simulink model "lab3"  (R2019b)
settings: Solver=FixedStepAuto  StartTime=0.0  StopTime=100.0  RelTol=1e-3
settings Model: Creator=Michał  LastModifiedBy=Michał

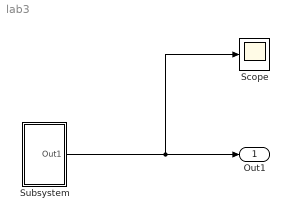
== system lab3 ==
  Scope : Scope
  Subsystem : Subsystem  mask{m=10, l=3, k=1, g=10, phi=90, phi0=0}
      mask prompts: m "masa"; l "dlugosc"; k "tlumienie"
  Out1 : Outport
  wires:
  Subsystem/1(Out1) -> Scope/1, Out1/1

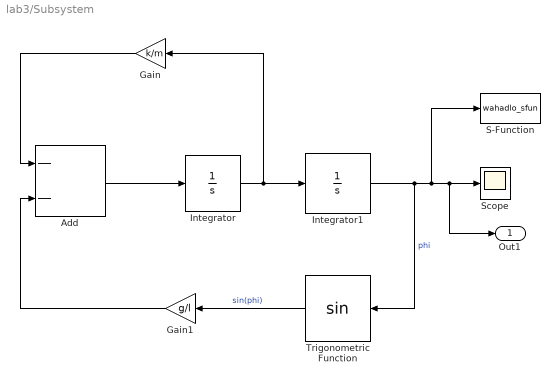
== system lab3/Subsystem ==
  Add : Sum  Inputs=--
  Gain : Gain  Gain=k/m
  Gain1 : Gain  Gain=g/l
  Integrator : Integrator  InitialCondition=phi * pi/180
  Integrator1 : Integrator  InitialCondition=phi0 * pi/180
  S-Function : S-Function  FunctionName=wahadlo_sfun  Parameters=l,m,phi0  SFunctionDeploymentMode=off  EnableBusSupport=off
  Scope : Scope
  Trigonometric Function : Trigonometry
  Out1 : Outport
  wires:
  Integrator1/1 -> Trigonometric Function/1, S-Function/1, Out1/1, Scope/1  "phi"
  Integrator/1 -> Gain/1, Integrator1/1
  Add/1 -> Integrator/1
  Gain/1 -> Add/1
  Trigonometric Function/1 -> Gain1/1  "sin(phi)"
  Gain1/1 -> Add/2
